simulink model "simulation_nonlinear_WT_toggle_Lab"  (R2023a)
settings: Solver=VariableStepAuto  StartTime=0.0  StopTime=inf  RelTol=1e-3
values from neighbouring files (symbols this model uses):
  a_1 = 0.048    [Preperatory_WT_Lab.m]
  a_2 = 0.0497    [Preperatory_WT_Lab.m]
  A_t = 50*1e-4    (= 0.005)    [Preperatory_WT_Lab.m]
  initial = [h1_0 h2_0]'    [Preperatory_WT_Lab.m]
  Kd = 55    [Preperatory_WT_Lab.m]
  Ki = 1.4    [Preperatory_WT_Lab.m]
  Kp = 70    [Preperatory_WT_Lab.m]
undefined symbols (not defined in the file or in its folder): d_w, K_pump, National_Instruments, PCI, u_max
libraries: sldrtlib x3, simulink x1, slpidlib x1
settings Model: Creator=EAL  LastModifiedBy=EAL

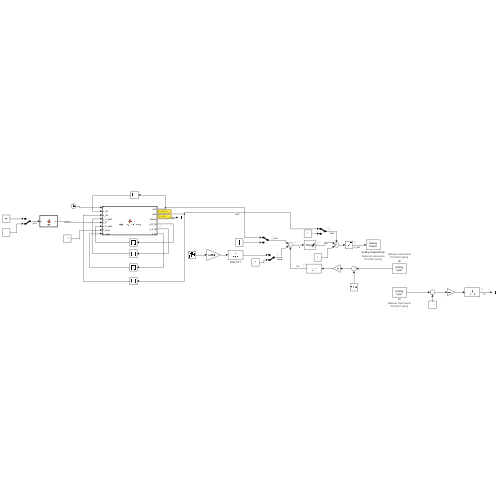
[thumbnail: Simulink's stored preview of the top-level diagram]
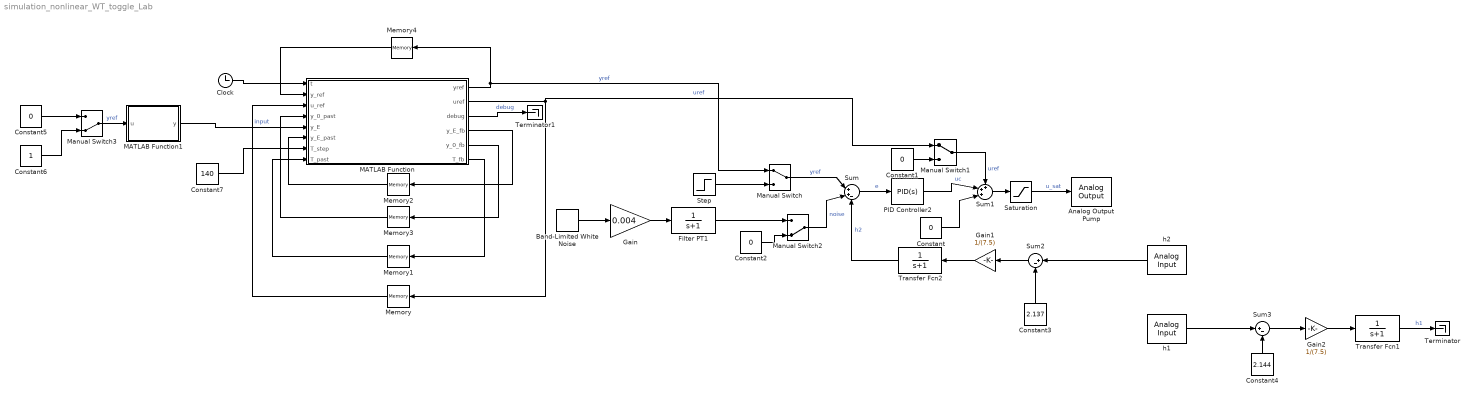
== system simulation_nonlinear_WT_toggle_Lab ==
  Analog Output Pump : sldrtlib/Analog Output  SampleTime=0.1  MaxMissedTicks=10  ShowMissedTicks=off  YieldWhenWaiting=off  DrvName=National_Instruments/PCI-6221  DrvAddress=4294967295  DrvOptions=[0 0 0 0 0]  Channels=1  RangeMode=1  VoltRange=1  InitialValue=[]  FinalValue=[]
      settings: AttributesFormatString=National Instruments\nPCI-6221 [auto]
  Band-Limited White Noise : simulink/Sources/Band-Limited White Noise  Cov=[0.1]  Ts=0.1  seed=[23341]
  Clock : Clock
  Constant{,1..2,5} (4 alike) : Constant  Value=0
  Constant3 : Constant  Value=2.137
  Constant4 : Constant  Value=2.144
  Constant6 : Constant
  Constant7 : Constant  Value=140
  Filter PT1 : TransferFcn  Denominator=[1 1]
  Gain : Gain  Gain=0.004
  Gain1 : Gain  Gain=1/(7.5)
  Gain2 : Gain  Gain=1/(7.5)
  MATLAB Function : MATLAB Function  TreatAsAtomicUnit=on
  MATLAB Function1 : MATLAB Function  TreatAsAtomicUnit=on
  Manual Switch : ManualSwitch
  Manual Switch1 : ManualSwitch
  Manual Switch2 : ManualSwitch  CurrentSetting=0
  Manual Switch3 : ManualSwitch  CurrentSetting=0
  Memory : Memory
  Memory1 : Memory
  Memory2 : Memory
  Memory3 : Memory  InitialCondition=initial(1)
  Memory4 : Memory  InitialCondition=initial(1)
  PID Controller2 : slpidlib/PID Controller  Controller=PID  Form=Parallel  TimeDomain=Continuous-time  UseExternalTs=off  SampleTime=-1  IntegratorMethod=Forward Euler  FilterMethod=Forward Euler  ControllerParametersSource=internal  P=Kp  I=Ki  UseKiTs=off  D=Kd  N=100  UseFilter=on  TunerSelectOption=Transfer Function Based (PID Tuner App)  InitialConditionSource=internal  InitialConditionForIntegrator=0  InitialConditionForFilter=0  DifferentiatorICPrevScaledInput=0  ExternalReset=none  TrackingMode=off  Kt=1  LimitOutput=on  SatLimitsSource=internal  UpperSaturationLimit=inf  LowerSaturationLimit=-inf  LinearizeAsGain=on  AntiWindupMode=clamping  Kb=1  LimitIntegrator=off  UpperIntegratorSaturationLimit=inf  LowerIntegratorSaturationLimit=-inf  POutMin=[]  POutMax=[]  IOutMin=[]  IOutMax=[]  DOutMin=[]  DOutMax=[]  NOutMin=[]  NOutMax=[]  SumOutMin=[]  SumOutMax=[]  SaturationOutMin=[]  SaturationOutMax=[]  PParamMin=[]  PParamMax=[]  IParamMin=[]  IParamMax=[]  DParamMin=[]  DParamMax=[]  NParamMin=[]  NParamMax=[]  KbParamMin=[]  KbParamMax=[]  KtParamMin=[]  KtParamMax=[]  KbOutMin=[]  KbOutMax=[]  KtOutMin=[]  KtOutMax=[]  IntegratorOutMin=[]  IntegratorOutMax=[]  FilterOutMin=[]  FilterOutMax=[]  SumI1OutMin=[]  SumI1OutMax=[]  SumI2OutMin=[]  SumI2OutMax=[]  SumI3OutMin=[]  SumI3OutMax=[]  SumI4OutMin=[]  SumI4OutMax=[]  SumDOutMin=[]  SumDOutMax=[]  DifferentiatorOutMin=[]  DifferentiatorOutMax=[]  FilterDiffOutCoefMin=[]  FilterDiffOutCoefMax=[]  ReciprocalOutMin=[]  ReciprocalOutMax=[]  SumDenOutMin=[]  SumDenOutMax=[]  SumNumOutMin=[]  SumNumOutMax=[]  DivideOutMin=[]  DivideOutMax=[]  UdiffTsProdOutMin=[]  UdiffTsProdOutMax=[]  NTsProdOutMin=[]  NTsProdOutMax=[]  UintegralTsProdOutMin=[]  UintegralTsProdOutMax=[]  UngainTsProdOutMin=[]  UngainTsProdOutMax=[]  ClampingZeroOutDataTypeStr=Inherit: Inherit via back propagation  ClampingZeroOutMin=[]  ClampingZeroOutMax=[]  FilterDenConstantOutDataTypeStr=Inherit: Inherit via back propagation  FilterDenConstantOutMin=[]  FilterDenConstantOutMax=[]  PCopyOutDataTypeStr=Inherit: Inherit via back propagation  PCopyOutMin=[]  PCopyOutMax=[]  NCopyOutDataTypeStr=Inherit: Inherit via back propagation  NCopyOutMin=[]  NCopyOutMax=[]  IntegratorContinuousStateAttributes=''  IntegratorStateMustResolveToSignalObject=off  IntegratorRTWStateStorageClass=Auto  FilterContinuousStateAttributes=''  FilterStateMustResolveToSignalObject=off  FilterRTWStateStorageClass=Auto  ParallelPVariant=InternalParameters  IdealPVariant=Disabled  IVariant=InternalParameters  DVariant=InternalParameters  IntegratorVariant=Continuous  SatVariant=Enabled  AWVariant=ContClampingParallel  PCopyVariant=Disabled  TRVariant=Disabled  FdbkBlocksVariant=Forward  IdealPFdbkVariant=Disabled  SatFdbkVariant=Disabled  DerivativeFilterVariant=ContFilter  NVariant=InternalParameters  NCopyVariant=Disabled  FilterICVariant=InternalICsFilter  IntegratorICVariant=InternalICs  ExternalResetVariant=Disabled  TRSumVariant=Passthrough  SumFdbkVariant=Disabled  SumVariant=Sum_PID  TsampFilterVariant=InternalTs  TsampNgainVariant=Passthrough  TsampIntegralVariant=Disabled_SignalSpec  ExternalSaturationOutDataTypeStr=Inherit: Same as second input
  Saturation : Saturate  UpperLimit=u_max  LowerLimit=0
  Step : Step  After=0.08  SampleTime=0
  Sum : Sum  Inputs=|++-
  Sum1 : Sum  Inputs=+++|
  Sum2 : Sum  Inputs=|+-
  Sum3 : Sum  Inputs=|+-
  Terminator : Terminator
  Terminator1 : Terminator
  Transfer Fcn1 : TransferFcn  Denominator=[1 1]
  Transfer Fcn2 : TransferFcn  Denominator=[1 1]
  h1 : sldrtlib/Analog Input  SampleTime=0.1  MaxMissedTicks=10  ShowMissedTicks=off  YieldWhenWaiting=off  DrvName=National_Instruments/PCI-6221  DrvAddress=4294967295  DrvOptions=[0 0 0 0 0]  Channels=1  RangeMode=1  VoltRange=2  DataType=1
      settings: AttributesFormatString=National Instruments\nPCI-6221 [auto]
  h2 : sldrtlib/Analog Input  SampleTime=0.1  MaxMissedTicks=10  ShowMissedTicks=off  YieldWhenWaiting=off  DrvName=National_Instruments/PCI-6221  DrvAddress=4294967295  DrvOptions=[0 0 0 0 0]  Channels=2  RangeMode=1  VoltRange=2  DataType=1
      settings: AttributesFormatString=National Instruments\nPCI-6221 [auto]
  wires:
  Gain1/1 -> Transfer Fcn2/1
  Constant/1 -> Sum1/3
  Sum3/1 -> Gain2/1
  h2/1 -> Sum2/1
  Saturation/1 -> Analog Output Pump/1  "u_sat"
  Transfer Fcn2/1 -> Sum/3  "h2"
  Constant2/1 -> Manual Switch2/2
  h1/1 -> Sum3/1
  Transfer Fcn1/1 -> Terminator/1  "h1"
  Gain2/1 -> Transfer Fcn1/1
  Manual Switch2/1 -> Sum/2  "noise"
  Manual Switch1/1 -> Sum1/1  "uref"
  Sum2/1 -> Gain1/1
  Step/1 -> Manual Switch/2
  Constant3/1 -> Sum2/2
  Sum1/1 -> Saturation/1
  Filter PT1/1 -> Manual Switch2/1
  PID Controller2/1 -> Sum1/2  "uc"
  Gain/1 -> Filter PT1/1
  Sum/1 -> PID Controller2/1  "e"
  Manual Switch/1 -> Sum/1  "yref"
  Band-Limited White Noise/1 -> Gain/1
  Constant1/1 -> Manual Switch1/2
  Constant4/1 -> Sum3/2
  MATLAB Function/2(uref) -> Manual Switch1/1, Memory/1  "uref"
  Constant6/1 -> Manual Switch3/2
  Memory3/1 -> MATLAB Function/4(y_0_past)
  Memory2/1 -> MATLAB Function/6(y_E_past)
  MATLAB Function/4(y_E_fb) -> Memory2/1
  Constant5/1 -> Manual Switch3/1
  MATLAB Function/5(y_0_fb) -> Memory3/1
  Manual Switch3/1 -> MATLAB Function1/1(u)  "yref"
  Memory4/1 -> MATLAB Function/2(y_ref)
  Memory1/1 -> MATLAB Function/8(T_past)
  MATLAB Function/6(T_fb) -> Memory1/1
  Memory/1 -> MATLAB Function/3(u_ref)
  Constant7/1 -> MATLAB Function/7(T_step)
  MATLAB Function/3(debug) -> Terminator1/1  "debug"
  MATLAB Function/1(yref) -> Manual Switch/1, Memory4/1  "yref"
  Clock/1 -> MATLAB Function/1(t)
  MATLAB Function1/1(y) -> MATLAB Function/5(y_E)  "input"

== matlab function simulation_nonlinear_WT_toggle_Lab/MATLAB Function ==
  data: yref output; uref output; t input; y_ref input; u_ref input; y_0_past input; y_E input; y_E_past input; T_step input; T_past input; d_w parameter; A_t parameter; K_pump parameter; debug output; y_E_fb output; y_0_fb output; T_fb output; a_1 parameter; a_2 parameter
function [yref, uref, debug, y_E_fb, y_0_fb, T_fb] = trajectory_planning(t, y_ref, u_ref, y_0_past, y_E, y_E_past, T_step, T_past,d_w, A_t, K_pump,a_1, a_2)
    % t: Current simulation time
    % y_0: Initial height of the ball
    % y_T: Desired height of the ball
    % T: Duration of the trajectory
    % tau_w: Fan time constant
    % a3, a2, a1: System coefficients
    % k_w: Fan gain

   

    % Order of the system
    n = 2;

    if(y_E == y_E_past) % still in the same transition
        y_0 = y_0_past;
    else    % start of new transition
        y_0 = y_ref;
        T_past = t;
    end
    
     % Normalize the current time
    tau = (t-T_past) / T_step;
    
    if(t < T_past + T_step)
        % Initialize coefficient matrix
        phi = zeros(n+1, 2*n+2);
    
        % Fill the first row of the coefficient matrix
        for k = 0:n
        phi(1,n+1-k) = nchoosek(n,k)*(-1)^k/(n+k+1);
        end
        
        % Add factor (which is multiplied by the sum) to all coefficients
        phi = factorial(2*n+1)/factorial(n)^2*phi;
        
        for j = 1:n
        phi(j+1,j+1:end) = 1/T_step*polyder(phi(j,j:end));
        end
        
        phi4 = zeros(n+1,length(tau));
        
        for i = 1:n+1
            phi4(i,:) = polyval(phi(i,:),tau);
        end
        
        % Compute the scaled trajectory
        yf = (y_E - y_0) * phi4;
        yf(1) = y_0 + yf(1); % Add the initial height for the non-derived function
    
        % Compute the angular velocity and its derivative

        y_h1 = yf(2,:).*yf(2,:)/(a_1)^2+(a_2)^2*yf(1,:)/(a_1)^2;
        y_h1_dot= 2*(yf(2,:)/a_1+sqrt(yf(1,:))).*(yf(3,:)/a_1+1./(2*sqrt(yf(1,:))).*yf(2,:));
        
        uref=(y_h1_dot + a_1*sqrt(y_h1))*d_w*A_t/K_pump;
        
        % Output the current reference trajectory and control input
        yref = yf(1);
        debug = phi4(1);
    else
        uref = u_ref;
        yref = y_ref;
        debug = 0;
    end
    T_fb = T_past;
    y_0_fb = y_0;
    y_E_fb = y_E;
    
end

== matlab function simulation_nonlinear_WT_toggle_Lab/MATLAB Function1 ==
  data: u input; y output
function y = fcn(u)

if(u)
    y = 0.04;
else
    y = 0.08;
end
